simulink subsystem "EnergyElectric"  (R2023b)
settings: Solver=VariableStepAuto  StartTime=0.0  StopTime=10.0  RelTol=1e-3
settings Model: Creator=jjha  LastModifiedBy=jjha

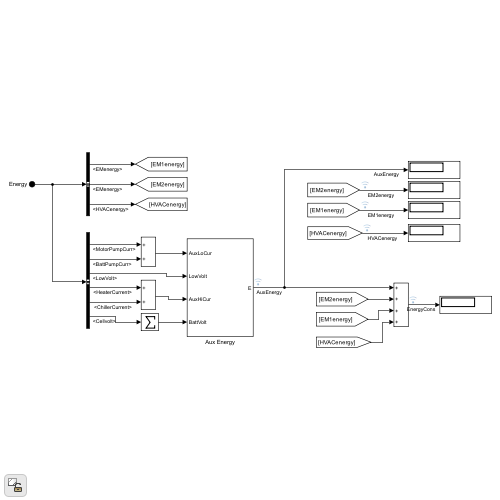
[thumbnail: Simulink's stored preview of the top-level diagram]
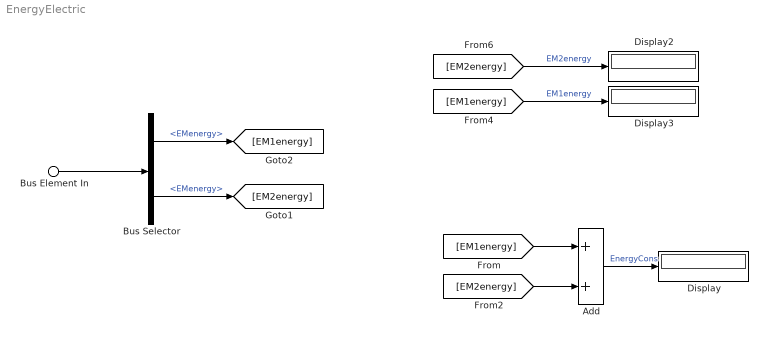
== system EnergyElectric ==
  Bus Element In : Inport  PortName=Energy
  Add : Sum
  Bus Selector : BusSelector  OutputSignals=M1.EMenergy,M2.EMenergy
  Display : Display
  Display2 : Display
  Display3 : Display
  wires:
  [EM2energy] -> Add/2
  [EM1energy] -> Add/1
  Add/1 -> Display/1  "EnergyCons"
  [EM2energy] -> Display2/1  "EM2energy"
  [EM1energy] -> Display3/1  "EM1energy"
  Bus Element In/1 -> Bus Selector/1
  Bus Selector/2 -> [EM2energy]  "<EMenergy>"
  Bus Selector/1 -> [EM1energy]  "<EMenergy>"
